simulink model "add_fft"  (R2020a)
settings: Solver=VariableStepAuto  StartTime=0.0  StopTime=25600  RelTol=1e-3
libraries: hdlsllib x4, dsphdlxfrm x1
settings Model: Creator=sunip  LastModifiedBy=sunip
settings OptimizationCC: BlockReduction=off  ConditionallyExecuteInputs=off  DefaultParameterBehavior=Inlined  SimCompilerOptimization=on
settings DebuggingCC: AlgebraicLoopMsg=error
settings HardwareCC: ProdBitPerPointer=32  ProdBitPerSizeT=32  ProdBitPerPtrDiffT=32  ProdLargestAtomicFloat=None  ProdIntDivRoundTo=Undefined  ProdEndianess=Unspecified  ProdWordSize=32  ProdHWDeviceType=ASIC/FPGA->ASIC/FPGA  TargetBitPerLong=64  TargetBitPerPointer=64  TargetBitPerSizeT=64  TargetBitPerPtrDiffT=64  TargetLongLongMode=on  TargetIntDivRoundTo=Zero  TargetEndianess=LittleEndian  TargetWordSize=64  TargetHWDeviceType=Custom Processor->MATLAB Host Computer  ProdEqTarget=off

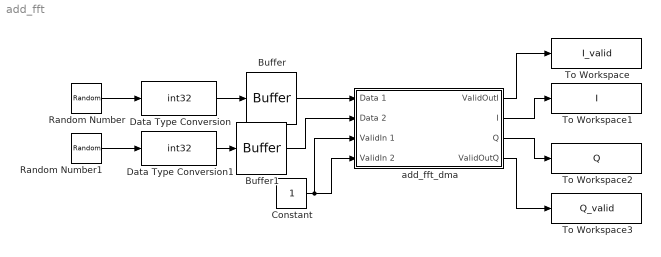
== system add_fft ==
  Buffer : Buffer  N=256  OutputFrames=off
  Buffer1 : Buffer  N=256  OutputFrames=off
  Constant : Constant  OutDataTypeStr=boolean
  Data Type Conversion : DataTypeConversion  OutDataTypeStr=int32
  Data Type Conversion1 : DataTypeConversion  OutDataTypeStr=int32
  Random Number : RandomNumber  Mean=10  SampleTime=100
  Random Number1 : RandomNumber  Mean=10  SampleTime=100
  To Workspace : ToWorkspace  VariableName=I_valid  SaveFormat=Timeseries  SampleTime=-1
  To Workspace1 : ToWorkspace  VariableName=I  SaveFormat=Timeseries  SampleTime=-1
  To Workspace2 : ToWorkspace  VariableName=Q  SaveFormat=Timeseries  SampleTime=-1
  To Workspace3 : ToWorkspace  VariableName=Q_valid  SaveFormat=Timeseries  SampleTime=-1
  add_fft_dma : Subsystem  TreatAsAtomicUnit=on
  wires:
  Constant/1 -> add_fft_dma/3(ValidIn 1), add_fft_dma/4(ValidIn 2)
  add_fft_dma/1(ValidOutI) -> To Workspace/1
  Random Number/1 -> Data Type Conversion/1
  Data Type Conversion1/1 -> Buffer1/1
  add_fft_dma/2(I) -> To Workspace1/1
  Data Type Conversion/1 -> Buffer/1
  Random Number1/1 -> Data Type Conversion1/1
  add_fft_dma/4(ValidOutQ) -> To Workspace3/1
  add_fft_dma/3(Q) -> To Workspace2/1
  Buffer/1 -> add_fft_dma/1(Data 1)
  Buffer1/1 -> add_fft_dma/2(Data 2)

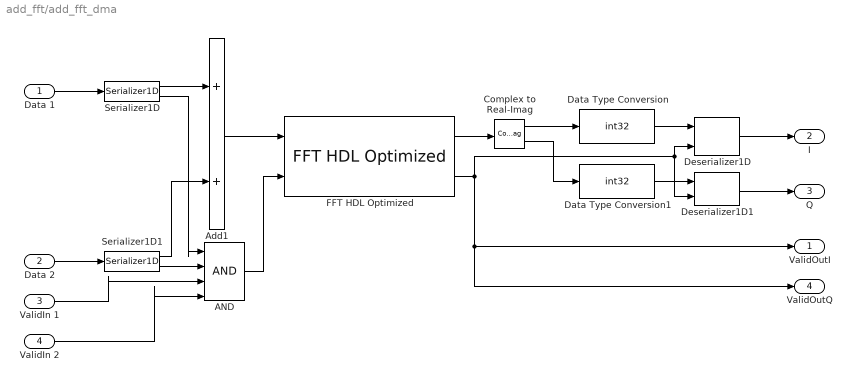
== system add_fft/add_fft_dma ==
  Data 1 : Inport  OutDataTypeStr=int32  SampleTime=100
  Data 2 : Inport  Port=2  OutDataTypeStr=int32  SampleTime=100
  ValidIn 1 : Inport  Port=3
  ValidIn 2 : Inport  Port=4
  AND : Logic  Inputs=4  IconShape=distinctive  AllPortsSameDT=off  OutDataTypeStr=boolean
  Add1 : Sum
  Complex to Real-Imag : ComplexToRealImag
  Data Type Conversion : DataTypeConversion  OutDataTypeStr=int32
  Data Type Conversion1 : DataTypeConversion  OutDataTypeStr=int32
  Deserializer1D : hdlsllib/HDL Operations/Deserializer1D  Ratio=1  IdleCycles=0  InitialCondition=0  startIn=off  validIn=on  validOut=off  inputDataDimensions=-1  inputSampleTime=-1  inputSignalType=auto
      settings: SourceProductBaseCode=SL
  Deserializer1D1 : hdlsllib/HDL Operations/Deserializer1D  Ratio=1  IdleCycles=0  InitialCondition=0  startIn=off  validIn=on  validOut=off  inputDataDimensions=-1  inputSampleTime=-1  inputSignalType=auto
      settings: SourceProductBaseCode=SL
  FFT HDL Optimized : dsphdlxfrm/FFT HDL Optimized  FFTLength=256  Architecture=Streaming Radix 2^2  ComplexMultiplication=Use 4 multipliers and 2 adders  BitReversedOutput=on  BitReversedInput=off  Normalize=off  SimulateUsing=Code generation  RoundingMethod=Floor  ResetInputPort=off  StartOutputPort=off  EndOutputPort=off
      settings: SourceProductBaseCode=DS
  Serializer1D : hdlsllib/HDL Operations/Serializer1D  Ratio=1  IdleCycles=0  validIn=off  startOut=off  validOut=on  inputDataDimensions=-1  inputSampleTime=-1  inputSignalType=auto
      settings: SourceProductBaseCode=SL
  Serializer1D1 : hdlsllib/HDL Operations/Serializer1D  Ratio=1  IdleCycles=0  validIn=off  startOut=off  validOut=on  inputDataDimensions=-1  inputSampleTime=-1  inputSignalType=auto
      settings: SourceProductBaseCode=SL
  ValidOutI : Outport
  I : Outport  Port=2
  Q : Outport  Port=3
  ValidOutQ : Outport  Port=4
  wires:
  ValidIn 1/1 -> AND/3
  Complex to Real-Imag/2 -> Data Type Conversion1/1
  Data Type Conversion/1 -> Deserializer1D/1
  Data Type Conversion1/1 -> Deserializer1D1/1
  Deserializer1D1/1 -> Q/1
  FFT HDL Optimized/1 -> Complex to Real-Imag/1
  FFT HDL Optimized/2 -> Deserializer1D1/2, Deserializer1D/2, ValidOutQ/1, ValidOutI/1
  Data 2/1 -> Serializer1D1/1
  Serializer1D1/2 -> AND/2
  ValidIn 2/1 -> AND/4
  AND/1 -> FFT HDL Optimized/2
  Serializer1D/1 -> Add1/1
  Serializer1D/2 -> AND/1
  Add1/1 -> FFT HDL Optimized/1
  Data 1/1 -> Serializer1D/1
  Deserializer1D/1 -> I/1
  Serializer1D1/1 -> Add1/2
  Complex to Real-Imag/1 -> Data Type Conversion/1
